simulink model "drone_dynamics_completed"  (R2025a)
settings: Solver=VariableStepAuto  StartTime=0.0  StopTime=10.0  RelTol=1e-3
settings Model: Creator=romai  LastModifiedBy=yasmi

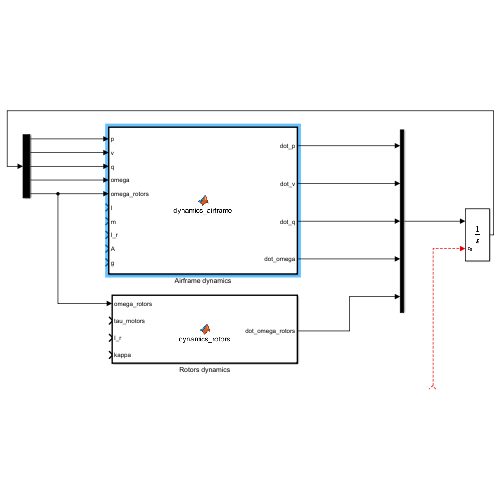
[thumbnail: Simulink's stored preview of the top-level diagram]
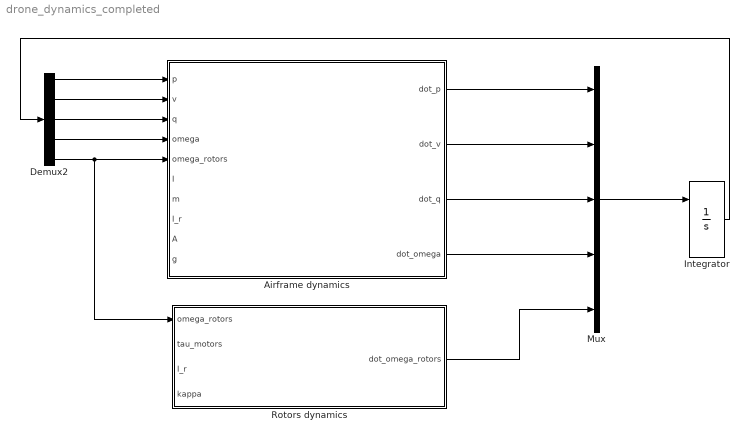
== system drone_dynamics_completed ==
  Airframe dynamics : MATLAB Function  TreatAsAtomicUnit=on
  Demux2 : Demux  Outputs=[3, 3, 4, 3, 4]
  Integrator : Integrator  InitialConditionSource=external
  Mux : Mux  Inputs=5
  Rotors dynamics : MATLAB Function  TreatAsAtomicUnit=on
  wires:
  ? -> Integrator/2
  Rotors dynamics/1(dot_omega_rotors) -> Mux/5
  Airframe dynamics/1(dot_p) -> Mux/1
  Demux2/5 -> Rotors dynamics/1(omega_rotors), Airframe dynamics/5(omega_rotors)
  Demux2/2 -> Airframe dynamics/2(v)
  Mux/1 -> Integrator/1
  Airframe dynamics/4(dot_omega) -> Mux/4
  Airframe dynamics/2(dot_v) -> Mux/2
  Integrator/1 -> Demux2/1
  Airframe dynamics/3(dot_q) -> Mux/3
  Demux2/3 -> Airframe dynamics/3(q)
  Demux2/1 -> Airframe dynamics/1(p)
  Demux2/4 -> Airframe dynamics/4(omega)

== matlab function drone_dynamics_completed/Rotors dynamics ==
  data: omega_rotors input; tau_motors input; I_r input; dot_omega_rotors output; kappa input
function dot_omega_rotors  = dynamics_rotors(omega_rotors, tau_motors, I_r, kappa)
    % DYNAMICS_ROTORS Computes the time derivative of the angular velocities of the rotors.
    %
    % Inputs:
    %      Time varying state variables:
    %   omega_rotors - Angular velocities of the rotors (4-vector)
    %   tau_motors   - Torques generated by the motors (4-vector)
    %
    %      Constant parameters:
    %   I_r          - Single rotor rotational inertia with respect to its axis of rotation (scalar)
    %   kappa        - ?whats it called? (scalar) 
    %
    % Outputs:
    %   dot_omega_rotors  - Time derivative of the angular velocities of
    %   the rotors (4-vector)


   
    drag_rotors = kappa * omega_rotors .^ 2;
    dot_omega_rotors = tau_motors / I_r - drag_rotors

end

% Manque I_r et Kappa = coeff de trainée

== matlab function drone_dynamics_completed/Airframe dynamics ==
  data: p input; dot_p output; v input; dot_v output; q input; omega input; omega_rotors input; I input; m input; I_r input; A input; g input; dot_q output; dot_omega output
function [dot_p, dot_v, dot_q, dot_omega] = dynamics_airframe(...
    p,v,q,omega, ...            % state
    omega_rotors,I,m,I_r,A,g)   % parameters

    % DYNAMICS_AIRFRAME Computes the time derivative of the state (p,v,q,omega) of the drone's airframe.
    %
    % Inputs:
    %      Time varying state variables:
    %   p            - Position (3-vector)
    %   v            - Velocity (3-vector)
    %   q            - Orientation (4-vector to be interpreted as a unit quaternion)
    %   omega        - Angular velocity (3-vector)
    %   omega_rotors - Angular velocities of the rotors (4-vector)
    %
    %      Constant parameters:
    %   I            - Rotational inertia matrix of the drone (3x3 matrix)
    %   m            - Mass of the airframe (scalar)
    %   I_r          - Single rotor rotational inertia with respect to its axis of rotation (scalar)
    %   A            - Matrix relating (squared) rotor angular velocities to thrust and torques (4x4 matrix)
    %   g            - Gravitational acceleration, positive (scalar)
    %
    % Outputs:
    %   dot_p        - Time derivative of position (3-vector)
    %   dot_v        - Time derivative of velocity (3-vector)
    %   dot_q        - Time derivative of orientation (4-vector to be interpreted as a quaternion in T_q(S^3))
    %   dot_omega    - Time derivative of angular velocity (in body frame) (3-vector)

    q = quaternion(q);  % simulink doesn't support quaternion signals.
    omega_rotors_2 = omega_rotors .^ 2;  % (proportional to the lifts generated by the rotors)

    % Thrust and (rigid body) torques.
    T = A(1,:) * omega_rotors_2;
    tau_a = A(2:4,:) * omega_rotors_2; % (in body frame)

    % Gyroscopic effect.
    G_a = I_r * sum(omega_rotors) * [omega(2), -omega(1), 0];

    % Airframe dynamics.
    dot_p = v;
    dot_v = [0,0,-g] + T/m * rotatepoint(q, [0,0,1]);
    dot_q = q * quaternion([0, 0.5 * omega]);
    dot_omega = I \ (tau_a + G_a - cross(omega, I * omega));

    dot_q = compact(dot_q).'; % simulink doesn't support quaternion signals.

    % Constants 
    m = 1.3 % Mass of the drone (kg)
    I = [0.02, 0, 0; 0, 0.02, 0; 0, 0, 0.04]; % Inertia Matrix 
    l = 0.275; % Distance from the center to each rotor (m)
    g = 9.81;  % Gravitational acceleration (m/s^2)

    c_T = 7.8e-6; % Thrust coefficient 
    c_D = 1.1e-7;  % Drag coefficient (N. rad.s^2.kg^(-1))
   

    % Matrix A 
    A = [c_T, c_T, c_T, c_T;   % Total thrust
    0, l * c_T, 0, -l * c_T;  % Roll torque
    -l * c_T, 0, l * c_T, 0;  % Pitch torque
    c_D, -c_D, c_D, -c_D];  % Yaw torque
